simulink library "Brakes_Axle3_PedalAbstract_DiscDiscDisc"  (R2025a)
settings: Solver=VariableStepAuto  StartTime=0.0  StopTime=10.0  RelTol=1e-3
undefined symbols (not defined in the file): Brakes
libraries: Brakes_Elements x6, sdl_lib x6, fl_lib x6, nesl_utility x6
Description:
  | Component of Simscape Vehicle Templates Library
  | 
  | Copyright 2018-2025 The MathWorks, Inc.
settings Model: Creator=smiller  LastModifiedBy=smiller
settings SolverCC: AlgebraicLoopSolver=TrustRegion
settings DataIOCC: ReturnWorkspaceOutputs=off
settings OptimizationCC: ReuseModelBlockBuffer=off
settings DebuggingCC: UnconnectedInputMsg=warning  UnconnectedOutputMsg=warning  UnconnectedLineMsg=warning  ArithmeticOperatorsInVariantConditions=warning
settings ModelReferenceCC: EnableRefExpFcnMdlSchedulingChecks=on
settings SFSimCC: CustomCodeUndefinedFunction=UseInterfaceOnly
settings RTWCC: GPUComputeCapability=3.5  DLArmComputeVersion=19.05

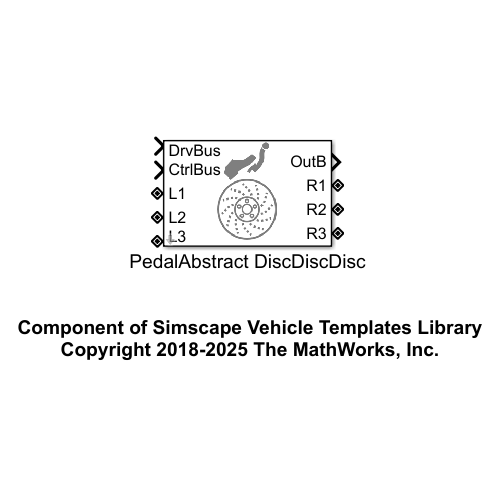
[thumbnail: Simulink's stored preview of the top-level diagram]
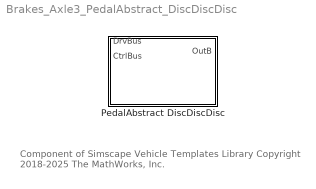
== system Brakes_Axle3_PedalAbstract_DiscDiscDisc ==
  note: Component of Simscape Vehicle Templates Library
      | Copyright 2018-2025 The MathWorks, Inc.
  PedalAbstract DiscDiscDisc : Subsystem  Tag=PublishSubsystem  VariantControl=Pedal  mask(Disc Brakes, Pedal Input){brk_pad_rad_a1=Brakes.Axle1.DiscAndPad.lMeanRadius.Value, brk_pad_rad_a2=Brakes.Axle2.DiscAndPad.lMeanRadius.Value, brk_pad_rad_a3=Brakes.Axle3.DiscAndPad.lMeanRadius.Value, brk_cyl_bore_a1=Brakes.Axle1.Caliper.lCylinderDiameter.Value, brk_cyl_bore_a2=Brakes.Axle2.Caliper.lCylinderDiameter.Value, brk_cyl_bore_a3=Brakes.Axle3.Caliper.lCylinderDiameter.Value, brk_n_pads_a1=Brakes.Axle1.DiscAndPad.NPads.Value, brk_n_pads_a2=Brakes.Axle2.DiscAndPad.NPads.Value, brk_n_pads_a3=Brakes.Axle3.DiscAndPad.NPads.Value, brk_mu_static_a1=Brakes.Axle1.DiscAndPad.rMuStatic.Value, brk_mu_static_a2=Brakes.Axle2.DiscAndPad.rMuStatic.Value, brk_mu_static_a3=Brakes.Axle3.DiscAndPad.rMuStatic.Value, brk_mu_kin_a1=Brakes.Axle1.DiscAndPad.rMuKinetic.Value, brk_mu_kin_a2=Brakes.Axle2.DiscAndPad.rMuKinetic.Value, brk_mu_kin_a3=Brakes.Axle3.DiscAndPad.rMuKinetic.Value, brk_trans_vel_a1=Brakes.Axle1.DiscAndPad.nTransition.Value, brk_trans_vel_a2=Brakes.Axle2.DiscAndPad.nTransition.Value, brk_trans_vel_a3=Brakes.Axle3.DiscAndPad.nTransition.Value, brk_visc_coef_a1=Brakes.Axle1.DiscAndPad.dViscous.Value, brk_visc_coef_a2=Brakes.Axle2.DiscAndPad.dViscous.Value, brk_visc_coef_a3=Brakes.Axle3.DiscAndPad.dViscous.Value, brk_max_p_a1=Brakes.Axle1.Caliper.pMax.Value, brk_max_p_a2=Brakes.Axle2.Caliper.pMax.Value, brk_max_p_a3=Brakes.Axle3.Caliper.pMax.Value, brk_filt_a1=1/Brakes.Axle1.Caliper.fActuatorCutoff.Value, brk_filt_a2=1/Brakes.Axle2.Caliper.fActuatorCutoff.Value, brk_filt_a3=1/Brakes.Axle3.Caliper.fActuatorCutoff.Value}
      mask help: Model braking system with disc brakes for three axles. Takes brake pedal travel as input, actuator dynamics modeled as a transfer function.
      mask TypeOptions brk_pad_rad_a1: Disc Brake L1/r_mean | Disc Brake R1/r_mean
      mask TypeOptions brk_pad_rad_a2: Disc Brake L2/r_mean | Disc Brake R2/r_mean
      mask TypeOptions brk_pad_rad_a3: Disc Brake L3/r_mean | Disc Brake R3/r_mean
      mask TypeOptions brk_cyl_bore_a1: Disc Brake L1/bore | Disc Brake R1/bore
      mask TypeOptions brk_cyl_bore_a2: Disc Brake L2/bore | Disc Brake R2/bore
      mask TypeOptions brk_cyl_bore_a3: Disc Brake L3/bore | Disc Brake R3/bore
      mask TypeOptions brk_n_pads_a1: Disc Brake L1/n_pads | Disc Brake R1/n_pads
      mask TypeOptions brk_n_pads_a2: Disc Brake L2/n_pads | Disc Brake R2/n_pads
      mask TypeOptions brk_n_pads_a3: Disc Brake L3/n_pads | Disc Brake R3/n_pads
      mask TypeOptions brk_mu_static_a1: Disc Brake L1/mu_static | Disc Brake R1/mu_static
      mask TypeOptions brk_mu_static_a2: Disc Brake L2/mu_static | Disc Brake R2/mu_static
      mask TypeOptions brk_mu_static_a3: Disc Brake L3/mu_static | Disc Brake R3/mu_static
      mask TypeOptions brk_mu_kin_a1: Disc Brake L1/mu_coulomb | Disc Brake R1/mu_coulomb
      mask TypeOptions brk_mu_kin_a2: Disc Brake L2/mu_coulomb | Disc Brake R2/mu_coulomb
      mask TypeOptions brk_mu_kin_a3: Disc Brake L3/mu_coulomb | Disc Brake R3/mu_coulomb
      mask TypeOptions brk_trans_vel_a1: Disc Brake L1/brkwy_vel | Disc Brake R1/brkwy_vel
      mask TypeOptions brk_trans_vel_a2: Disc Brake L2/brkwy_vel | Disc Brake R2/brkwy_vel
      mask TypeOptions brk_trans_vel_a3: Disc Brake L3/brkwy_vel | Disc Brake R3/brkwy_vel
      mask TypeOptions brk_visc_coef_a1: Disc Brake L1/visc_coef | Disc Brake R1/visc_coef
      mask TypeOptions brk_visc_coef_a2: Disc Brake L2/visc_coef | Disc Brake R2/visc_coef
      mask TypeOptions brk_visc_coef_a3: Disc Brake L3/visc_coef | Disc Brake R3/visc_coef
      mask TypeOptions brk_max_p_a1: Actuator L1/brk_max_p | Actuator R1/brk_max_p
      mask TypeOptions brk_max_p_a2: Actuator L2/brk_max_p | Actuator R2/brk_max_p
      mask TypeOptions brk_max_p_a3: Actuator L3/brk_max_p | Actuator R3/brk_max_p
      mask TypeOptions brk_filt_a1: Actuator L1/brk_filt | Actuator R1/brk_filt
      mask TypeOptions brk_filt_a2: Actuator L2/brk_filt | Actuator R2/brk_filt
      mask TypeOptions brk_filt_a3: Actuator L3/brk_filt | Actuator R3/brk_filt
      mask DialogControl cont_brakes Prompt: Brakes
      mask DialogControl cont_brk_geom Prompt: Geometry
      mask DialogControl text_brakes_a1 Prompt: Axle 1
      mask DialogControl text_brakes_a2 Prompt: Axle 2
      mask DialogControl text_brakes_a3 Prompt: Axle 3
      mask DialogControl text_brakes_pad_rad Prompt: Mean Pad Radius (m)
      mask DialogControl text_brakes_cyl_bore Prompt: Cylinder Bore (m)
      mask DialogControl text_brakes_n_pads Prompt: Number of pads
      mask DialogControl cont_brk_frict Prompt: Friction
      mask DialogControl text_brakes_mu_static Prompt: Static Coeff. (0-1)
      mask DialogControl text_brakes_mu_kin Prompt: Kinetic Coeff. (0-1)
      mask DialogControl text_brakes_trans_vel Prompt: Trans. Velocity (rad/s)
      mask DialogControl text_brakes_visc_coef Prompt: Viscous (N*m/(rad/s))
      mask DialogControl cont_brk_act Prompt: Actuator
      mask DialogControl text_brakes_maxp Prompt: Max Pad Pressure (Pa)
      mask DialogControl text_brakes_filt Prompt: Time Constant (s)
      mask Display: image('sm_car_vehicle_brakes_pedal_IMAGE.png');

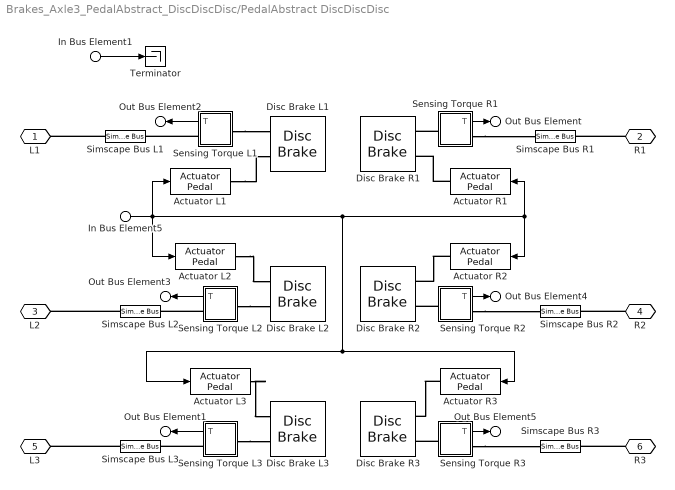
== system Brakes_Axle3_PedalAbstract_DiscDiscDisc/PedalAbstract DiscDiscDisc ==
  In Bus Element5 : Inport  PortName=DrvBus  Element=rBrakePedal
  In Bus Element1 : Inport  Port=2  PortName=CtrlBus
  Actuator L1 : Brakes_Elements/Actuator Pedal  brk_max_p=brk_max_p_a1  brk_filt=brk_filt_a1
  Actuator L2 : Brakes_Elements/Actuator Pedal  brk_max_p=brk_max_p_a2  brk_filt=brk_filt_a2
  Actuator L3 : Brakes_Elements/Actuator Pedal  brk_max_p=brk_max_p_a3  brk_filt=brk_filt_a3
  Actuator R1 : Brakes_Elements/Actuator Pedal  brk_max_p=brk_max_p_a1  brk_filt=brk_filt_a1
  Actuator R2 : Brakes_Elements/Actuator Pedal  brk_max_p=brk_max_p_a2  brk_filt=brk_filt_a2
  Actuator R3 : Brakes_Elements/Actuator Pedal  brk_max_p=brk_max_p_a3  brk_filt=brk_filt_a3
  Disc Brake L1 : sdl_lib/Brakes & Detents/Rotational/Disc Brake  r_mean=brk_pad_rad_a1 m  bore=brk_cyl_bore_a1 m  n_pads=brk_n_pads_a1  thermal_port=simscape.enum.thermaleffects.omit  mu_static=brk_mu_static_a1  mu_coulomb=brk_mu_kin_a1  temperature_TLU=[280, 300, 320] K  mu_static_TLU=[.9, .8, .7]  mu_coulomb_TLU=[.8, .7, .6]  brkwy_vel=brk_trans_vel_a1 rad/s  visc_coef=brk_visc_coef_a1 N*m/(rad/s)  thermal_mass=50 kJ/K  temperature_specify=off  temperature_priority=High  temperature=300 K  temperature_nominal_specify=off  temperature_nominal_value=1  temperature_nominal_unit=K
  Disc Brake L2 : sdl_lib/Brakes & Detents/Rotational/Disc Brake  r_mean=brk_pad_rad_a2 m  bore=brk_cyl_bore_a2 m  n_pads=brk_n_pads_a2  thermal_port=simscape.enum.thermaleffects.omit  mu_static=brk_mu_static_a2  mu_coulomb=brk_mu_kin_a2  temperature_TLU=[280, 300, 320] K  mu_static_TLU=[.9, .8, .7]  mu_coulomb_TLU=[.8, .7, .6]  brkwy_vel=brk_trans_vel_a2 rad/s  visc_coef=brk_visc_coef_a2 N*m/(rad/s)  thermal_mass=50 kJ/K  temperature_specify=off  temperature_priority=High  temperature=300 K  temperature_nominal_specify=off  temperature_nominal_value=1  temperature_nominal_unit=K
  Disc Brake L3 : sdl_lib/Brakes & Detents/Rotational/Disc Brake  r_mean=brk_pad_rad_a3 m  bore=brk_cyl_bore_a3 m  n_pads=brk_n_pads_a3  thermal_port=simscape.enum.thermaleffects.omit  mu_static=brk_mu_static_a3  mu_coulomb=brk_mu_kin_a3  temperature_TLU=[280, 300, 320] K  mu_static_TLU=[.9, .8, .7]  mu_coulomb_TLU=[.8, .7, .6]  brkwy_vel=brk_trans_vel_a3 rad/s  visc_coef=brk_visc_coef_a3 N*m/(rad/s)  thermal_mass=50 kJ/K  temperature_specify=off  temperature_priority=High  temperature=300 K  temperature_nominal_specify=off  temperature_nominal_value=1  temperature_nominal_unit=K
  Disc Brake R1 : sdl_lib/Brakes & Detents/Rotational/Disc Brake  r_mean=brk_pad_rad_a1 m  bore=brk_cyl_bore_a1 m  n_pads=brk_n_pads_a1  thermal_port=simscape.enum.thermaleffects.omit  mu_static=brk_mu_static_a1  mu_coulomb=brk_mu_kin_a1  temperature_TLU=[280, 300, 320] K  mu_static_TLU=[.9, .8, .7]  mu_coulomb_TLU=[.8, .7, .6]  brkwy_vel=brk_trans_vel_a1 rad/s  visc_coef=brk_visc_coef_a1 N*m/(rad/s)  thermal_mass=50 kJ/K  temperature_specify=off  temperature_priority=High  temperature=300 K  temperature_nominal_specify=off  temperature_nominal_value=1  temperature_nominal_unit=K
  Disc Brake R2 : sdl_lib/Brakes & Detents/Rotational/Disc Brake  r_mean=brk_pad_rad_a2 m  bore=brk_cyl_bore_a2 m  n_pads=brk_n_pads_a2  thermal_port=simscape.enum.thermaleffects.omit  mu_static=brk_mu_static_a2  mu_coulomb=brk_mu_kin_a2  temperature_TLU=[280, 300, 320] K  mu_static_TLU=[.9, .8, .7]  mu_coulomb_TLU=[.8, .7, .6]  brkwy_vel=brk_trans_vel_a2 rad/s  visc_coef=brk_visc_coef_a2 N*m/(rad/s)  thermal_mass=50 kJ/K  temperature_specify=off  temperature_priority=High  temperature=300 K  temperature_nominal_specify=off  temperature_nominal_value=1  temperature_nominal_unit=K
  Disc Brake R3 : sdl_lib/Brakes & Detents/Rotational/Disc Brake  r_mean=brk_pad_rad_a3 m  bore=brk_cyl_bore_a3 m  n_pads=brk_n_pads_a3  thermal_port=simscape.enum.thermaleffects.omit  mu_static=brk_mu_static_a3  mu_coulomb=brk_mu_kin_a3  temperature_TLU=[280, 300, 320] K  mu_static_TLU=[.9, .8, .7]  mu_coulomb_TLU=[.8, .7, .6]  brkwy_vel=brk_trans_vel_a3 rad/s  visc_coef=brk_visc_coef_a3 N*m/(rad/s)  thermal_mass=50 kJ/K  temperature_specify=off  temperature_priority=High  temperature=300 K  temperature_nominal_specify=off  temperature_nominal_value=1  temperature_nominal_unit=K
  Sensing Torque L1 : Subsystem
  Sensing Torque L2 : Subsystem
  Sensing Torque L3 : Subsystem
  Sensing Torque R1 : Subsystem
  Sensing Torque R2 : Subsystem
  Sensing Torque R3 : Subsystem
  Simscape Bus L1 : SimscapeBus  HierarchyStrings=Axle1D
  Simscape Bus L2 : SimscapeBus  HierarchyStrings=Axle1D
  Simscape Bus L3 : SimscapeBus  HierarchyStrings=Axle1D
  Simscape Bus R1 : SimscapeBus  HierarchyStrings=Axle1D
  Simscape Bus R2 : SimscapeBus  HierarchyStrings=Axle1D
  Simscape Bus R3 : SimscapeBus  HierarchyStrings=Axle1D
  Terminator : Terminator
  L1 : PMIOPort  Side=Left
  R1 : PMIOPort  Port=2  Side=Right
  L2 : PMIOPort  Port=3  Side=Left
  R2 : PMIOPort  Port=4  Side=Right
  L3 : PMIOPort  Port=5  Side=Left
  R3 : PMIOPort  Port=6  Side=Right
  Out Bus Element2 : Outport  VectorParamsAs1DForOutWhenUnconnected=off  PortName=OutB  Element=MBrakeL1
  Out Bus Element : Outport  VectorParamsAs1DForOutWhenUnconnected=off  PortName=OutB  Element=MBrakeR1
  Out Bus Element3 : Outport  VectorParamsAs1DForOutWhenUnconnected=off  PortName=OutB  Element=MBrakeL2
  Out Bus Element4 : Outport  VectorParamsAs1DForOutWhenUnconnected=off  PortName=OutB  Element=MBrakeR2
  Out Bus Element1 : Outport  VectorParamsAs1DForOutWhenUnconnected=off  PortName=OutB  Element=MBrakeL3
  Out Bus Element5 : Outport  VectorParamsAs1DForOutWhenUnconnected=off  PortName=OutB  Element=MBrakeR3
  wires:
  Sensing Torque R2/1(T) -> Out Bus Element4/1
  Sensing Torque L2/1(T) -> Out Bus Element3/1
  Sensing Torque R1/1(T) -> Out Bus Element/1
  Sensing Torque L1/1(T) -> Out Bus Element2/1
  In Bus Element1/1 -> Terminator/1
  In Bus Element5/1 -> Actuator L2/1, Actuator R2/1, Actuator R1/1, Actuator R3/1, Actuator L3/1, Actuator L1/1
  Sensing Torque L3/1(T) -> Out Bus Element1/1
  Sensing Torque R3/1(T) -> Out Bus Element5/1
  connections:
  Sensing Torque R2/RConn1 -- Simscape Bus R2/LConn1
  Sensing Torque L2/RConn1 -- Simscape Bus L2/LConn1
  Sensing Torque R1/RConn1 -- Simscape Bus R1/LConn1
  Sensing Torque L1/RConn1 -- Simscape Bus L1/LConn1
  Sensing Torque L1/LConn1 -- Disc Brake L1/LConn2
  Simscape Bus L1/RConn1 -- L1/RConn1
  Sensing Torque L2/LConn1 -- Disc Brake L2/LConn2
  Simscape Bus L2/RConn1 -- L2/RConn1
  R2/RConn1 -- Simscape Bus R2/RConn1
  R1/RConn1 -- Simscape Bus R1/RConn1
  Actuator R2/RConn1 -- Disc Brake R2/LConn1
  Actuator L1/RConn1 -- Disc Brake L1/LConn1
  Actuator L2/RConn1 -- Disc Brake L2/LConn1
  Actuator R1/RConn1 -- Disc Brake R1/LConn1
  Sensing Torque R1/LConn1 -- Disc Brake R1/LConn2
  Sensing Torque R2/LConn1 -- Disc Brake R2/LConn2
  Actuator R3/RConn1 -- Disc Brake R3/LConn1
  R3/RConn1 -- Simscape Bus R3/RConn1
  Actuator L3/RConn1 -- Disc Brake L3/LConn1
  Sensing Torque R3/LConn1 -- Disc Brake R3/LConn2
  Sensing Torque L3/RConn1 -- Simscape Bus L3/LConn1
  Simscape Bus L3/RConn1 -- L3/RConn1
  Sensing Torque R3/RConn1 -- Simscape Bus R3/LConn1
  Sensing Torque L3/LConn1 -- Disc Brake L3/LConn2

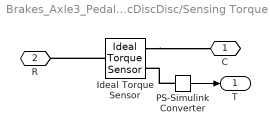
== system Brakes_Axle3_PedalAbstract_DiscDiscDisc/PedalAbstract DiscDiscDisc/Sensing Torque L1 ==
  Ideal Torque Sensor : fl_lib/Mechanical/Mechanical Sensors/Ideal Torque Sensor
  PS-Simulink Converter : nesl_utility/PS-Simulink Converter  PhysicalDomain=network_engine_domain  SubClassName=ps_output  LeftPortType=input  RightPortType=output  PseudoPeriodic=off  Frequencies=[]  VectorFormat=1-D array  Unit=N*m  AffineConversion=off
  C : PMIOPort  Side=Right
  R : PMIOPort  Port=2  Side=Left
  T : Outport  VectorParamsAs1DForOutWhenUnconnected=off
  wires:
  PS-Simulink Converter/1 -> T/1
  connections:
  Ideal Torque Sensor/LConn1 -- R/RConn1
  Ideal Torque Sensor/RConn1 -- C/RConn1
  PS-Simulink Converter/LConn1 -- Ideal Torque Sensor/RConn2

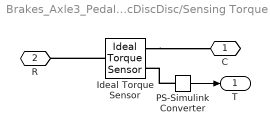
== system Brakes_Axle3_PedalAbstract_DiscDiscDisc/PedalAbstract DiscDiscDisc/Sensing Torque L2 ==
  Ideal Torque Sensor : fl_lib/Mechanical/Mechanical Sensors/Ideal Torque Sensor
  PS-Simulink Converter : nesl_utility/PS-Simulink Converter  PhysicalDomain=network_engine_domain  SubClassName=ps_output  LeftPortType=input  RightPortType=output  PseudoPeriodic=off  Frequencies=[]  VectorFormat=1-D array  Unit=N*m  AffineConversion=off
  C : PMIOPort  Side=Right
  R : PMIOPort  Port=2  Side=Left
  T : Outport  VectorParamsAs1DForOutWhenUnconnected=off
  wires:
  PS-Simulink Converter/1 -> T/1
  connections:
  Ideal Torque Sensor/LConn1 -- R/RConn1
  Ideal Torque Sensor/RConn1 -- C/RConn1
  PS-Simulink Converter/LConn1 -- Ideal Torque Sensor/RConn2

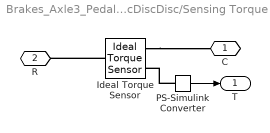
== system Brakes_Axle3_PedalAbstract_DiscDiscDisc/PedalAbstract DiscDiscDisc/Sensing Torque L3 ==
  Ideal Torque Sensor : fl_lib/Mechanical/Mechanical Sensors/Ideal Torque Sensor
  PS-Simulink Converter : nesl_utility/PS-Simulink Converter  PhysicalDomain=network_engine_domain  SubClassName=ps_output  LeftPortType=input  RightPortType=output  PseudoPeriodic=off  Frequencies=[]  VectorFormat=1-D array  Unit=N*m  AffineConversion=off
  C : PMIOPort  Side=Right
  R : PMIOPort  Port=2  Side=Left
  T : Outport  VectorParamsAs1DForOutWhenUnconnected=off
  wires:
  PS-Simulink Converter/1 -> T/1
  connections:
  PS-Simulink Converter/LConn1 -- Ideal Torque Sensor/RConn2
  Ideal Torque Sensor/RConn1 -- C/RConn1
  Ideal Torque Sensor/LConn1 -- R/RConn1

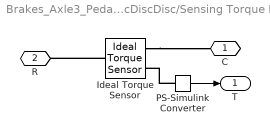
== system Brakes_Axle3_PedalAbstract_DiscDiscDisc/PedalAbstract DiscDiscDisc/Sensing Torque R1 ==
  Ideal Torque Sensor : fl_lib/Mechanical/Mechanical Sensors/Ideal Torque Sensor
  PS-Simulink Converter : nesl_utility/PS-Simulink Converter  PhysicalDomain=network_engine_domain  SubClassName=ps_output  LeftPortType=input  RightPortType=output  PseudoPeriodic=off  Frequencies=[]  VectorFormat=1-D array  Unit=N*m  AffineConversion=off
  C : PMIOPort  Side=Right
  R : PMIOPort  Port=2  Side=Left
  T : Outport  VectorParamsAs1DForOutWhenUnconnected=off
  wires:
  PS-Simulink Converter/1 -> T/1
  connections:
  PS-Simulink Converter/LConn1 -- Ideal Torque Sensor/RConn2
  Ideal Torque Sensor/RConn1 -- C/RConn1
  Ideal Torque Sensor/LConn1 -- R/RConn1

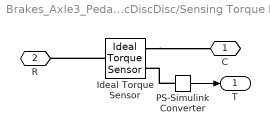
== system Brakes_Axle3_PedalAbstract_DiscDiscDisc/PedalAbstract DiscDiscDisc/Sensing Torque R2 ==
  Ideal Torque Sensor : fl_lib/Mechanical/Mechanical Sensors/Ideal Torque Sensor
  PS-Simulink Converter : nesl_utility/PS-Simulink Converter  PhysicalDomain=network_engine_domain  SubClassName=ps_output  LeftPortType=input  RightPortType=output  PseudoPeriodic=off  Frequencies=[]  VectorFormat=1-D array  Unit=N*m  AffineConversion=off
  C : PMIOPort  Side=Right
  R : PMIOPort  Port=2  Side=Left
  T : Outport  VectorParamsAs1DForOutWhenUnconnected=off
  wires:
  PS-Simulink Converter/1 -> T/1
  connections:
  PS-Simulink Converter/LConn1 -- Ideal Torque Sensor/RConn2
  Ideal Torque Sensor/RConn1 -- C/RConn1
  Ideal Torque Sensor/LConn1 -- R/RConn1

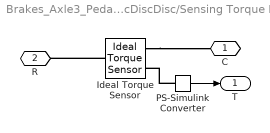
== system Brakes_Axle3_PedalAbstract_DiscDiscDisc/PedalAbstract DiscDiscDisc/Sensing Torque R3 ==
  Ideal Torque Sensor : fl_lib/Mechanical/Mechanical Sensors/Ideal Torque Sensor
  PS-Simulink Converter : nesl_utility/PS-Simulink Converter  PhysicalDomain=network_engine_domain  SubClassName=ps_output  LeftPortType=input  RightPortType=output  PseudoPeriodic=off  Frequencies=[]  VectorFormat=1-D array  Unit=N*m  AffineConversion=off
  C : PMIOPort  Side=Right
  R : PMIOPort  Port=2  Side=Left
  T : Outport  VectorParamsAs1DForOutWhenUnconnected=off
  wires:
  PS-Simulink Converter/1 -> T/1
  connections:
  Ideal Torque Sensor/LConn1 -- R/RConn1
  Ideal Torque Sensor/RConn1 -- C/RConn1
  PS-Simulink Converter/LConn1 -- Ideal Torque Sensor/RConn2
